simulink model "auto3exp"  (Simulink 8.2)
settings: Solver=ode4  StartTime=0.0  StopTime=10.0  RelTol=1e-3
settings Model: Creator=nathanlrf  LastModifiedBy=nathanlrf
settings DataIOCC: SignalLoggingSaveFormat=Dataset
settings OptimizationCC: ExpressionDepthLimit=128
settings DebuggingCC: FcnCallInpInsideContextMsg=EnableAllAsError  StateNameClashWarn=none
settings GRTTargetCC: CombineOutputUpdateFcns=on  GRTInterface=off

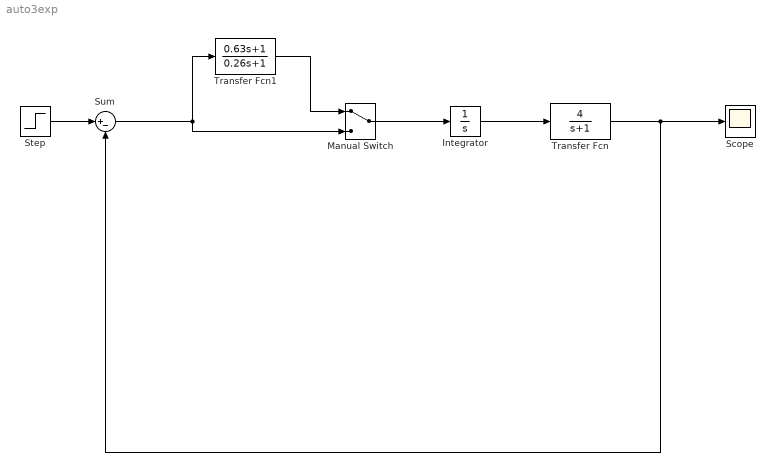
== system auto3exp ==
  Integrator : Integrator
  Manual Switch : ManualSwitch
  Scope : Scope
  Step : Step  SampleTime=0
  Sum : Sum  Inputs=|+-
  Transfer Fcn : TransferFcn  Numerator=4  Denominator=[1 1]
  Transfer Fcn1 : TransferFcn  Numerator=[0.63 1]  Denominator=[0.26 1]
  wires:
  Transfer Fcn1/1 -> Manual Switch/1
  Sum/1 -> Manual Switch/2, Transfer Fcn1/1
  Manual Switch/1 -> Integrator/1
  Integrator/1 -> Transfer Fcn/1
  Step/1 -> Sum/1
  Transfer Fcn/1 -> Sum/2, Scope/1
